simulink model "Copy_of_GNP"  (R2012b)
settings: Solver=ode3  StartTime=0.0  StopTime=sim_time  FixedStep=Ts  RelTol=1e-3
values from neighbouring files (symbols this model uses):
  education = 20    [simulate_gnp.m]
  food_effect_unit = 1    [simulate_gnp.m]
  food_employees = 20000    [simulate_gnp.m]
  food_material = 2    [simulate_gnp.m]
  food_price = 400    [simulate_gnp.m]
  food_production = 3    [simulate_gnp.m]
  food_salary = 15000    [simulate_gnp.m]
  oil_effect_unit = 15    [simulate_gnp.m]
  oil_employees = 5000    [simulate_gnp.m]
  oil_material = 10    [simulate_gnp.m]
  oil_price = 1000    [simulate_gnp.m]
  oil_production = 50    [simulate_gnp.m]
  oil_salary = 12000    [simulate_gnp.m]
  population = 100000    [simulate_gnp.m]
  public_average_salary = 25000    [simulate_gnp.m]
  public_employees = 20000    [simulate_gnp.m]
  tax = 0.3    [simulate_gnp.m]
  unemployees = (population - public_employees - car_employees -     oil_employees - food_employees)/population    (= 0.45)    [simulate_gnp.m]
undefined symbols (not defined in the file): car_employees, car_material, car_price, car_production, car_salary, KiEmployeeController
settings Model: Creator=ägarenn  LastModifiedBy=ägarenn
settings DebuggingCC: SolverPrmCheckMsg=none

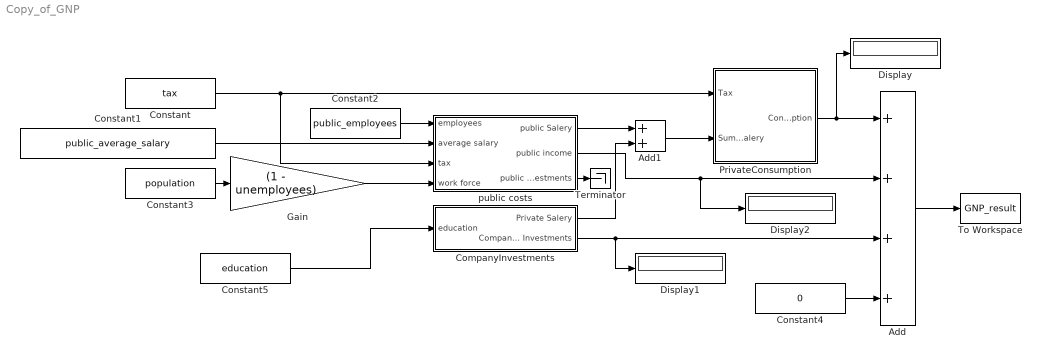
== system Copy_of_GNP ==
  Add : Sum  Inputs=++++
  Add1 : Sum
  CompanyInvestments : Subsystem
  Constant : Constant  Value=tax
  Constant1 : Constant  Value=public_average_salary
  Constant2 : Constant  Value=public_employees
  Constant3 : Constant  Value=population
  Constant4 : Constant  Value=0
  Constant5 : Constant  Value=education
  Display : Display
  Display1 : Display
  Display2 : Display
  Gain : Gain  Gain=(1 - unemployees)
  PrivateConsumption : Subsystem
  Terminator : Terminator
  To Workspace : ToWorkspace  VariableName=GNP_result  SampleTime=-1  SaveFormat=Timeseries
  public costs : Subsystem
  wires:
  Add/1 -> To Workspace/1
  CompanyInvestments/2(Company Investments) -> Display1/1, Add/3
  Add1/1 -> PrivateConsumption/2(SumSalery)
  public costs/1(public Salery) -> Add1/1
  CompanyInvestments/1(Private Salery) -> Add1/2
  public costs/2(public income) -> Display2/1, Add/2
  Constant/1 -> public costs/3(tax), PrivateConsumption/1(Tax)
  Constant1/1 -> public costs/2(average salary)
  Constant2/1 -> public costs/1(employees)
  Gain/1 -> public costs/4(work force)
  Constant3/1 -> Gain/1
  Constant4/1 -> Add/4
  public costs/3(public investments) -> Terminator/1
  PrivateConsumption/1(Consumption) -> Display/1, Add/1
  Constant5/1 -> CompanyInvestments/1(education)

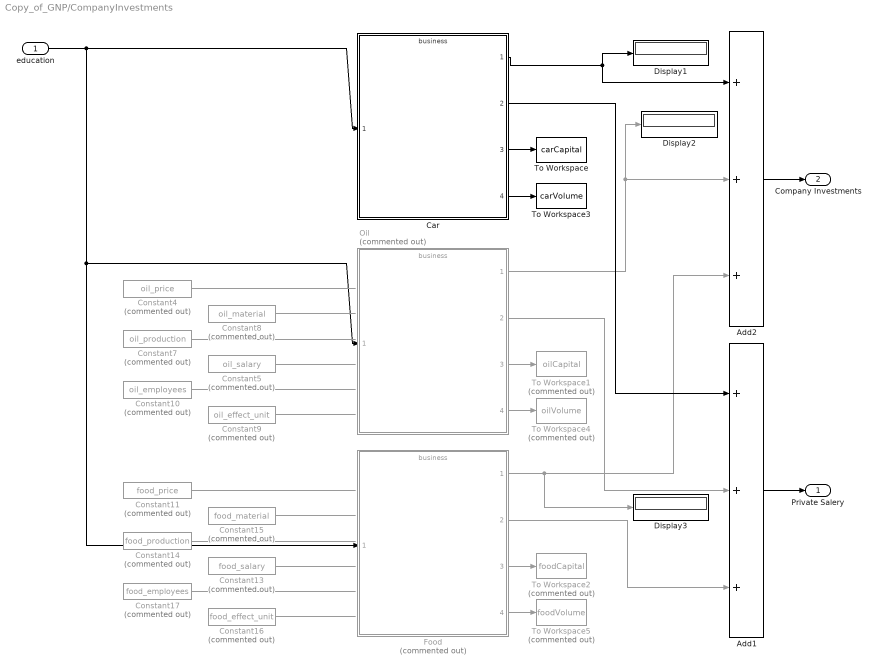
== system Copy_of_GNP/CompanyInvestments ==
  education : Inport
  Add1 : Sum  Inputs=+++
  Add2 : Sum  Inputs=+++
  Car : ModelReference  ModelNameDialog=business  SimulationMode=Normal  ModelReferenceVersion=1.45  CopyOfModelName=business  DefaultDataLogging=on  mask{price=car_price, material=car_material, producion=car_production, employees=car_employees, salary=car_salary, effect_unit=car_effect_unit, KpEmployeeController=KiEmployeeController, KiEmployeeController=KiEmployeeController}
      mask prompts: producion "production"; salary "salary_value"
      mask Display: image(imread('Images/factory.png'))
  Constant10 : Constant  Commented=on  Value=oil_employees
  Constant11 : Constant  Commented=on  Value=food_price
  Constant13 : Constant  Commented=on  Value=food_salary
  Constant14 : Constant  Commented=on  Value=food_production
  Constant15 : Constant  Commented=on  Value=food_material
  Constant16 : Constant  Commented=on  Value=food_effect_unit
  Constant17 : Constant  Commented=on  Value=food_employees
  Constant4 : Constant  Commented=on  Value=oil_price
  Constant5 : Constant  Commented=on  Value=oil_salary
  Constant7 : Constant  Commented=on  Value=oil_production
  Constant8 : Constant  Commented=on  Value=oil_material
  Constant9 : Constant  Commented=on  Value=oil_effect_unit
  Display1 : Display
  Display2 : Display
  Display3 : Display
  Food : ModelReference  Commented=on  ModelNameDialog=business  SimulationMode=Normal  ModelReferenceVersion=1.45  CopyOfModelName=business  DefaultDataLogging=on
  Oil : ModelReference  Commented=on  ModelNameDialog=business  SimulationMode=Normal  ModelReferenceVersion=1.45  CopyOfModelName=business  DefaultDataLogging=on
  To Workspace : ToWorkspace  VariableName=carCapital  SampleTime=-1  SaveFormat=Timeseries
  To Workspace1 : ToWorkspace  Commented=on  VariableName=oilCapital  SampleTime=-1  SaveFormat=Timeseries
  To Workspace2 : ToWorkspace  Commented=on  VariableName=foodCapital  SampleTime=-1  SaveFormat=Timeseries
  To Workspace3 : ToWorkspace  VariableName=carVolume  SampleTime=-1  SaveFormat=Timeseries
  To Workspace4 : ToWorkspace  Commented=on  VariableName=oilVolume  SampleTime=-1  SaveFormat=Timeseries
  To Workspace5 : ToWorkspace  Commented=on  VariableName=foodVolume  SampleTime=-1  SaveFormat=Timeseries
  Private Salery : Outport
  Company Investments : Outport  Port=2
  wires:
  Add2/1 -> Company Investments/1
  Car/1 -> Add2/1, Display1/1
  Oil/1 -> Add2/2, Display2/1
  Food/1 -> Display3/1, Add2/3
  Add1/1 -> Private Salery/1
  Car/2 -> Add1/1
  Oil/2 -> Add1/2
  Food/2 -> Add1/3
  education/1 -> Food/1, Oil/1, Car/1
  Constant4/1 -> ?
  Constant8/1 -> ?
  Constant7/1 -> ?
  Constant5/1 -> ?
  Constant10/1 -> ?
  Constant9/1 -> ?
  Constant11/1 -> ?
  Constant15/1 -> ?
  Constant14/1 -> ?
  Constant13/1 -> ?
  Constant17/1 -> ?
  Constant16/1 -> ?
  Car/3 -> To Workspace/1
  Oil/3 -> To Workspace1/1
  Food/3 -> To Workspace2/1
  Car/4 -> To Workspace3/1
  Oil/4 -> To Workspace4/1
  Food/4 -> To Workspace5/1

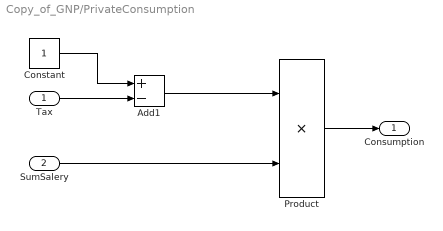
== system Copy_of_GNP/PrivateConsumption ==
  Tax : Inport
  SumSalery : Inport  Port=2
  Add1 : Sum  Inputs=+-
  Constant : Constant
  Product : Product  RndMeth=Zero
  Consumption : Outport
  wires:
  Product/1 -> Consumption/1
  Tax/1 -> Add1/2
  Add1/1 -> Product/1
  Constant/1 -> Add1/1
  SumSalery/1 -> Product/2

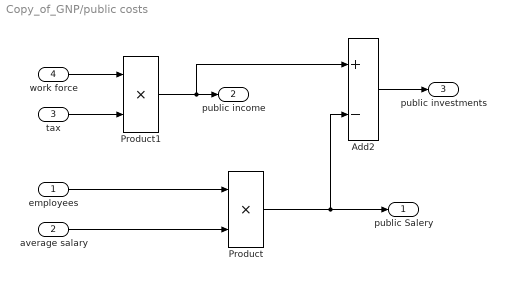
== system Copy_of_GNP/public costs ==
  employees : Inport
  average salary : Inport  Port=2
  tax : Inport  Port=3
  work force : Inport  Port=4
  Add2 : Sum  Inputs=+-
  Product : Product  RndMeth=Zero
  Product1 : Product  RndMeth=Zero
  public Salery : Outport
  public income : Outport  Port=2
  public investments : Outport  Port=3
  wires:
  Product/1 -> Add2/2, public Salery/1
  employees/1 -> Product/1
  average salary/1 -> Product/2
  work force/1 -> Product1/1
  tax/1 -> Product1/2
  Product1/1 -> Add2/1, public income/1
  Add2/1 -> public investments/1
